simulink model "Simulation_CHB_Gridconnected"  (R2023a)
settings: Solver=ode4  StartTime=0.0  StopTime=2  FixedStep=1e-6  RelTol=1e-3
libraries: spsMosfetLib x24, spsSeriesRLCBranchLib x9, spsVoltageMeasurementLib x9, spsControlledCurrentSourceLib x6, slpidlib x5, simulink x3, eePowerMeasurement x3, spsThreePhaseVIMeasurementLib x3, spsabctodq0Lib x2, spsStairGeneratorLib x1, spsPLL3phLib x1, spsThreePhaseSeriesRLCLoadLib x1
settings Model: Creator=Vigneshwaran R  LastModifiedBy=Vigneshwaran R

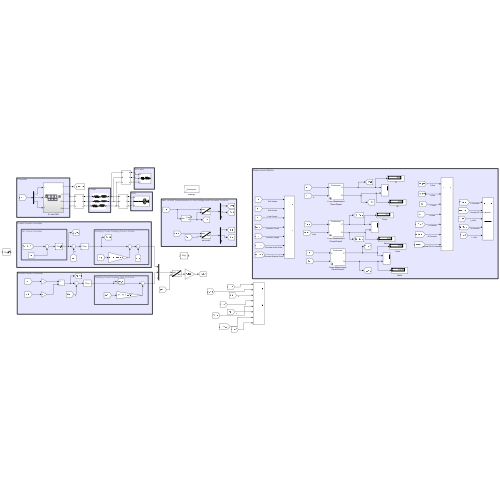
[thumbnail: Simulink's stored preview of the top-level diagram]
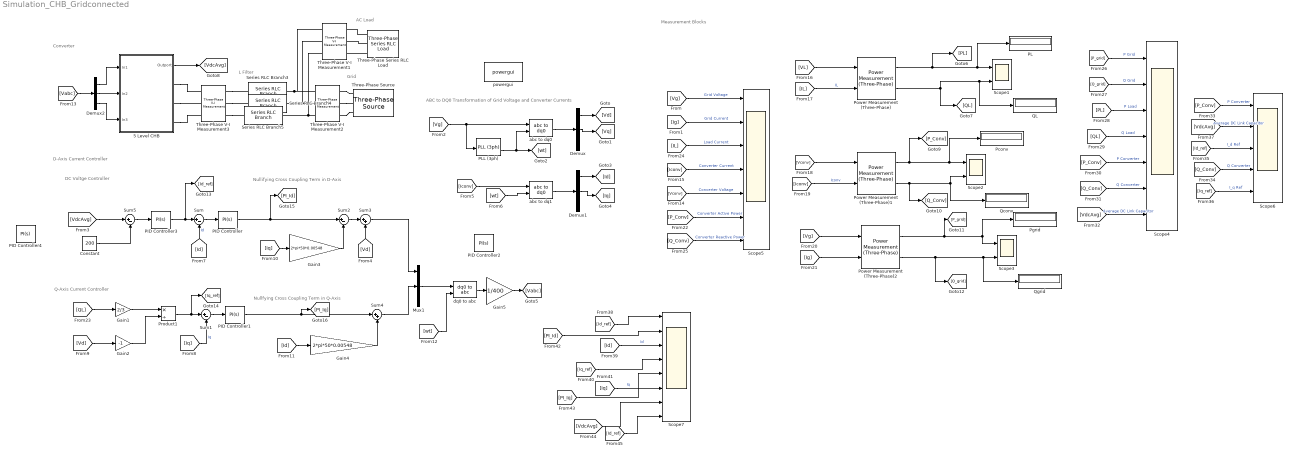
== system Simulation_CHB_Gridconnected ==
  note: Measurement Blocks
  note: L Filter
  note: D-Axis Current Controller
  note: Q-Axis Current Controller
  note: Nullfying Cross Coupling Term in Q-Axis
  note: Nullifying Cross Coupling Term in D-Axis
  note: DC Voltge Controller
  note: Grid
  note: AC Load
  note: ABC to DQ0 Transformation of Grid Voltage and Converter Currents
  note: Converter
  5 Level CHB : Subsystem
  Constant : Constant  Value=200
  Demux : Demux  Outputs=3
  Demux1 : Demux  Outputs=3
  Demux2 : Demux  Outputs=3
  Gain1 : Gain  Gain=2/3
  Gain2 : Gain  Gain=-1
  Gain3 : Gain  Gain=2*pi*50*0.00548
  Gain4 : Gain  Gain=2*pi*50*0.00548
  Gain5 : Gain  Gain=1/400
  Mux1 : Mux  Inputs=3
  PID Controller : slpidlib/PID Controller  Controller=PI  Form=Parallel  TimeDomain=Continuous-time  UseExternalTs=off  SampleTime=-1  IntegratorMethod=Forward Euler  FilterMethod=Forward Euler  ControllerParametersSource=internal  P=0.0847*400  I=1.577*400  UseKiTs=off  D=0  N=100  UseFilter=on  TunerSelectOption=Transfer Function Based (PID Tuner App)  InitialConditionSource=internal  InitialConditionForIntegrator=0  InitialConditionForFilter=0  DifferentiatorICPrevScaledInput=0  ExternalReset=none  TrackingMode=off  Kt=1  LimitOutput=off  SatLimitsSource=internal  UpperSaturationLimit=1  LowerSaturationLimit=-1  LinearizeAsGain=on  AntiWindupMode=none  Kb=1  LimitIntegrator=off  UpperIntegratorSaturationLimit=inf  LowerIntegratorSaturationLimit=-inf  POutMin=[]  POutMax=[]  IOutMin=[]  IOutMax=[]  DOutMin=[]  DOutMax=[]  NOutMin=[]  NOutMax=[]  SumOutMin=[]  SumOutMax=[]  SaturationOutMin=[]  SaturationOutMax=[]  PParamMin=[]  PParamMax=[]  IParamMin=[]  IParamMax=[]  DParamMin=[]  DParamMax=[]  NParamMin=[]  NParamMax=[]  KbParamMin=[]  KbParamMax=[]  KtParamMin=[]  KtParamMax=[]  KbOutMin=[]  KbOutMax=[]  KtOutMin=[]  KtOutMax=[]  IntegratorOutMin=[]  IntegratorOutMax=[]  FilterOutMin=[]  FilterOutMax=[]  SumI1OutMin=[]  SumI1OutMax=[]  SumI2OutMin=[]  SumI2OutMax=[]  SumI3OutMin=[]  SumI3OutMax=[]  SumI4OutMin=[]  SumI4OutMax=[]  SumDOutMin=[]  SumDOutMax=[]  DifferentiatorOutMin=[]  DifferentiatorOutMax=[]  FilterDiffOutCoefMin=[]  FilterDiffOutCoefMax=[]  ReciprocalOutMin=[]  ReciprocalOutMax=[]  SumDenOutMin=[]  SumDenOutMax=[]  SumNumOutMin=[]  SumNumOutMax=[]  DivideOutMin=[]  DivideOutMax=[]  UdiffTsProdOutMin=[]  UdiffTsProdOutMax=[]  NTsProdOutMin=[]  NTsProdOutMax=[]  UintegralTsProdOutMin=[]  UintegralTsProdOutMax=[]  UngainTsProdOutMin=[]  UngainTsProdOutMax=[]  ClampingZeroOutDataTypeStr=Inherit: Inherit via back propagation  ClampingZeroOutMin=[]  ClampingZeroOutMax=[]  FilterDenConstantOutDataTypeStr=Inherit: Inherit via back propagation  FilterDenConstantOutMin=[]  FilterDenConstantOutMax=[]  PCopyOutDataTypeStr=Inherit: Inherit via back propagation  PCopyOutMin=[]  PCopyOutMax=[]  NCopyOutDataTypeStr=Inherit: Inherit via back propagation  NCopyOutMin=[]  NCopyOutMax=[]  IntegratorContinuousStateAttributes=''  IntegratorStateMustResolveToSignalObject=off  IntegratorRTWStateStorageClass=Auto  FilterContinuousStateAttributes=''  FilterStateMustResolveToSignalObject=off  FilterRTWStateStorageClass=Auto  ParallelPVariant=InternalParameters  IdealPVariant=Disabled  IVariant=InternalParameters  DVariant=Disabled  IntegratorVariant=Continuous  SatVariant=Disabled  AWVariant=Passthrough  PCopyVariant=Disabled  TRVariant=Disabled  FdbkBlocksVariant=Forward  IdealPFdbkVariant=Disabled  SatFdbkVariant=Disabled  DerivativeFilterVariant=Disabled  NVariant=Disabled  NCopyVariant=Disabled_SignalSpec  FilterICVariant=Disabled  IntegratorICVariant=InternalICs  ExternalResetVariant=Disabled  TRSumVariant=Passthrough  SumFdbkVariant=Disabled  SumVariant=Sum_PI  TsampFilterVariant=InternalTs  TsampNgainVariant=Passthrough  TsampIntegralVariant=Disabled_SignalSpec  ExternalSaturationOutDataTypeStr=Inherit: Same as second input
  PID Controller1 : slpidlib/PID Controller  Controller=PI  Form=Parallel  TimeDomain=Continuous-time  UseExternalTs=off  SampleTime=-1  IntegratorMethod=Forward Euler  FilterMethod=Forward Euler  ControllerParametersSource=internal  P=0.0847*400  I=1.577*400  UseKiTs=off  D=0  N=100  UseFilter=on  TunerSelectOption=Transfer Function Based (PID Tuner App)  InitialConditionSource=internal  InitialConditionForIntegrator=0  InitialConditionForFilter=0  DifferentiatorICPrevScaledInput=0  ExternalReset=none  TrackingMode=off  Kt=1  LimitOutput=off  SatLimitsSource=internal  UpperSaturationLimit=1  LowerSaturationLimit=-1  LinearizeAsGain=on  AntiWindupMode=none  Kb=1  LimitIntegrator=off  UpperIntegratorSaturationLimit=inf  LowerIntegratorSaturationLimit=-inf  POutMin=[]  POutMax=[]  IOutMin=[]  IOutMax=[]  DOutMin=[]  DOutMax=[]  NOutMin=[]  NOutMax=[]  SumOutMin=[]  SumOutMax=[]  SaturationOutMin=[]  SaturationOutMax=[]  PParamMin=[]  PParamMax=[]  IParamMin=[]  IParamMax=[]  DParamMin=[]  DParamMax=[]  NParamMin=[]  NParamMax=[]  KbParamMin=[]  KbParamMax=[]  KtParamMin=[]  KtParamMax=[]  KbOutMin=[]  KbOutMax=[]  KtOutMin=[]  KtOutMax=[]  IntegratorOutMin=[]  IntegratorOutMax=[]  FilterOutMin=[]  FilterOutMax=[]  SumI1OutMin=[]  SumI1OutMax=[]  SumI2OutMin=[]  SumI2OutMax=[]  SumI3OutMin=[]  SumI3OutMax=[]  SumI4OutMin=[]  SumI4OutMax=[]  SumDOutMin=[]  SumDOutMax=[]  DifferentiatorOutMin=[]  DifferentiatorOutMax=[]  FilterDiffOutCoefMin=[]  FilterDiffOutCoefMax=[]  ReciprocalOutMin=[]  ReciprocalOutMax=[]  SumDenOutMin=[]  SumDenOutMax=[]  SumNumOutMin=[]  SumNumOutMax=[]  DivideOutMin=[]  DivideOutMax=[]  UdiffTsProdOutMin=[]  UdiffTsProdOutMax=[]  NTsProdOutMin=[]  NTsProdOutMax=[]  UintegralTsProdOutMin=[]  UintegralTsProdOutMax=[]  UngainTsProdOutMin=[]  UngainTsProdOutMax=[]  ClampingZeroOutDataTypeStr=Inherit: Inherit via back propagation  ClampingZeroOutMin=[]  ClampingZeroOutMax=[]  FilterDenConstantOutDataTypeStr=Inherit: Inherit via back propagation  FilterDenConstantOutMin=[]  FilterDenConstantOutMax=[]  PCopyOutDataTypeStr=Inherit: Inherit via back propagation  PCopyOutMin=[]  PCopyOutMax=[]  NCopyOutDataTypeStr=Inherit: Inherit via back propagation  NCopyOutMin=[]  NCopyOutMax=[]  IntegratorContinuousStateAttributes=''  IntegratorStateMustResolveToSignalObject=off  IntegratorRTWStateStorageClass=Auto  FilterContinuousStateAttributes=''  FilterStateMustResolveToSignalObject=off  FilterRTWStateStorageClass=Auto  ParallelPVariant=InternalParameters  IdealPVariant=Disabled  IVariant=InternalParameters  DVariant=Disabled  IntegratorVariant=Continuous  SatVariant=Disabled  AWVariant=Passthrough  PCopyVariant=Disabled  TRVariant=Disabled  FdbkBlocksVariant=Forward  IdealPFdbkVariant=Disabled  SatFdbkVariant=Disabled  DerivativeFilterVariant=Disabled  NVariant=Disabled  NCopyVariant=Disabled_SignalSpec  FilterICVariant=Disabled  IntegratorICVariant=InternalICs  ExternalResetVariant=Disabled  TRSumVariant=Passthrough  SumFdbkVariant=Disabled  SumVariant=Sum_PI  TsampFilterVariant=InternalTs  TsampNgainVariant=Passthrough  TsampIntegralVariant=Disabled_SignalSpec  ExternalSaturationOutDataTypeStr=Inherit: Same as second input
  PID Controller2 : slpidlib/PID Controller  Controller=PI  Form=Parallel  TimeDomain=Continuous-time  UseExternalTs=off  SampleTime=-1  IntegratorMethod=Forward Euler  FilterMethod=Forward Euler  ControllerParametersSource=internal  P=0.15  I=157.7  UseKiTs=off  D=0  N=100  UseFilter=on  TunerSelectOption=Transfer Function Based (PID Tuner App)  InitialConditionSource=internal  InitialConditionForIntegrator=0  InitialConditionForFilter=0  DifferentiatorICPrevScaledInput=0  ExternalReset=none  TrackingMode=off  Kt=1  LimitOutput=off  SatLimitsSource=internal  UpperSaturationLimit=1  LowerSaturationLimit=-1  LinearizeAsGain=on  AntiWindupMode=none  Kb=1  LimitIntegrator=off  UpperIntegratorSaturationLimit=inf  LowerIntegratorSaturationLimit=-inf  POutMin=[]  POutMax=[]  IOutMin=[]  IOutMax=[]  DOutMin=[]  DOutMax=[]  NOutMin=[]  NOutMax=[]  SumOutMin=[]  SumOutMax=[]  SaturationOutMin=[]  SaturationOutMax=[]  PParamMin=[]  PParamMax=[]  IParamMin=[]  IParamMax=[]  DParamMin=[]  DParamMax=[]  NParamMin=[]  NParamMax=[]  KbParamMin=[]  KbParamMax=[]  KtParamMin=[]  KtParamMax=[]  KbOutMin=[]  KbOutMax=[]  KtOutMin=[]  KtOutMax=[]  IntegratorOutMin=[]  IntegratorOutMax=[]  FilterOutMin=[]  FilterOutMax=[]  SumI1OutMin=[]  SumI1OutMax=[]  SumI2OutMin=[]  SumI2OutMax=[]  SumI3OutMin=[]  SumI3OutMax=[]  SumI4OutMin=[]  SumI4OutMax=[]  SumDOutMin=[]  SumDOutMax=[]  DifferentiatorOutMin=[]  DifferentiatorOutMax=[]  FilterDiffOutCoefMin=[]  FilterDiffOutCoefMax=[]  ReciprocalOutMin=[]  ReciprocalOutMax=[]  SumDenOutMin=[]  SumDenOutMax=[]  SumNumOutMin=[]  SumNumOutMax=[]  DivideOutMin=[]  DivideOutMax=[]  UdiffTsProdOutMin=[]  UdiffTsProdOutMax=[]  NTsProdOutMin=[]  NTsProdOutMax=[]  UintegralTsProdOutMin=[]  UintegralTsProdOutMax=[]  UngainTsProdOutMin=[]  UngainTsProdOutMax=[]  ClampingZeroOutDataTypeStr=Inherit: Inherit via back propagation  ClampingZeroOutMin=[]  ClampingZeroOutMax=[]  FilterDenConstantOutDataTypeStr=Inherit: Inherit via back propagation  FilterDenConstantOutMin=[]  FilterDenConstantOutMax=[]  PCopyOutDataTypeStr=Inherit: Inherit via back propagation  PCopyOutMin=[]  PCopyOutMax=[]  NCopyOutDataTypeStr=Inherit: Inherit via back propagation  NCopyOutMin=[]  NCopyOutMax=[]  IntegratorContinuousStateAttributes=''  IntegratorStateMustResolveToSignalObject=off  IntegratorRTWStateStorageClass=Auto  FilterContinuousStateAttributes=''  FilterStateMustResolveToSignalObject=off  FilterRTWStateStorageClass=Auto  ParallelPVariant=InternalParameters  IdealPVariant=Disabled  IVariant=InternalParameters  DVariant=Disabled  IntegratorVariant=Continuous  SatVariant=Disabled  AWVariant=Passthrough  PCopyVariant=Disabled  TRVariant=Disabled  FdbkBlocksVariant=Forward  IdealPFdbkVariant=Disabled  SatFdbkVariant=Disabled  DerivativeFilterVariant=Disabled  NVariant=Disabled  NCopyVariant=Disabled_SignalSpec  FilterICVariant=Disabled  IntegratorICVariant=InternalICs  ExternalResetVariant=Disabled  TRSumVariant=Passthrough  SumFdbkVariant=Disabled  SumVariant=Sum_PI  TsampFilterVariant=InternalTs  TsampNgainVariant=Passthrough  TsampIntegralVariant=Disabled_SignalSpec  ExternalSaturationOutDataTypeStr=Inherit: Same as second input
  PID Controller3 : slpidlib/PID Controller  Controller=PI  Form=Parallel  TimeDomain=Continuous-time  UseExternalTs=off  SampleTime=-1  IntegratorMethod=Forward Euler  FilterMethod=Forward Euler  ControllerParametersSource=internal  P=1*10  I=5*10  UseKiTs=off  D=0  N=100  UseFilter=on  TunerSelectOption=Transfer Function Based (PID Tuner App)  InitialConditionSource=internal  InitialConditionForIntegrator=0  InitialConditionForFilter=0  DifferentiatorICPrevScaledInput=0  ExternalReset=none  TrackingMode=off  Kt=1  LimitOutput=on  SatLimitsSource=internal  UpperSaturationLimit=200  LowerSaturationLimit=-200  LinearizeAsGain=on  AntiWindupMode=none  Kb=1  LimitIntegrator=off  UpperIntegratorSaturationLimit=inf  LowerIntegratorSaturationLimit=-inf  POutMin=[]  POutMax=[]  IOutMin=[]  IOutMax=[]  DOutMin=[]  DOutMax=[]  NOutMin=[]  NOutMax=[]  SumOutMin=[]  SumOutMax=[]  SaturationOutMin=[]  SaturationOutMax=[]  PParamMin=[]  PParamMax=[]  IParamMin=[]  IParamMax=[]  DParamMin=[]  DParamMax=[]  NParamMin=[]  NParamMax=[]  KbParamMin=[]  KbParamMax=[]  KtParamMin=[]  KtParamMax=[]  KbOutMin=[]  KbOutMax=[]  KtOutMin=[]  KtOutMax=[]  IntegratorOutMin=[]  IntegratorOutMax=[]  FilterOutMin=[]  FilterOutMax=[]  SumI1OutMin=[]  SumI1OutMax=[]  SumI2OutMin=[]  SumI2OutMax=[]  SumI3OutMin=[]  SumI3OutMax=[]  SumI4OutMin=[]  SumI4OutMax=[]  SumDOutMin=[]  SumDOutMax=[]  DifferentiatorOutMin=[]  DifferentiatorOutMax=[]  FilterDiffOutCoefMin=[]  FilterDiffOutCoefMax=[]  ReciprocalOutMin=[]  ReciprocalOutMax=[]  SumDenOutMin=[]  SumDenOutMax=[]  SumNumOutMin=[]  SumNumOutMax=[]  DivideOutMin=[]  DivideOutMax=[]  UdiffTsProdOutMin=[]  UdiffTsProdOutMax=[]  NTsProdOutMin=[]  NTsProdOutMax=[]  UintegralTsProdOutMin=[]  UintegralTsProdOutMax=[]  UngainTsProdOutMin=[]  UngainTsProdOutMax=[]  ClampingZeroOutDataTypeStr=Inherit: Inherit via back propagation  ClampingZeroOutMin=[]  ClampingZeroOutMax=[]  FilterDenConstantOutDataTypeStr=Inherit: Inherit via back propagation  FilterDenConstantOutMin=[]  FilterDenConstantOutMax=[]  PCopyOutDataTypeStr=Inherit: Inherit via back propagation  PCopyOutMin=[]  PCopyOutMax=[]  NCopyOutDataTypeStr=Inherit: Inherit via back propagation  NCopyOutMin=[]  NCopyOutMax=[]  IntegratorContinuousStateAttributes=''  IntegratorStateMustResolveToSignalObject=off  IntegratorRTWStateStorageClass=Auto  FilterContinuousStateAttributes=''  FilterStateMustResolveToSignalObject=off  FilterRTWStateStorageClass=Auto  ParallelPVariant=InternalParameters  IdealPVariant=Disabled  IVariant=InternalParameters  DVariant=Disabled  IntegratorVariant=Continuous  SatVariant=Enabled  AWVariant=Passthrough  PCopyVariant=Disabled  TRVariant=Disabled  FdbkBlocksVariant=Forward  IdealPFdbkVariant=Disabled  SatFdbkVariant=Disabled  DerivativeFilterVariant=Disabled  NVariant=Disabled  NCopyVariant=Disabled_SignalSpec  FilterICVariant=Disabled  IntegratorICVariant=InternalICs  ExternalResetVariant=Disabled  TRSumVariant=Passthrough  SumFdbkVariant=Disabled  SumVariant=Sum_PI  TsampFilterVariant=InternalTs  TsampNgainVariant=Passthrough  TsampIntegralVariant=Disabled_SignalSpec  ExternalSaturationOutDataTypeStr=Inherit: Same as second input
  PID Controller4 : slpidlib/PID Controller  Controller=PI  Form=Parallel  TimeDomain=Continuous-time  UseExternalTs=off  SampleTime=-1  IntegratorMethod=Forward Euler  FilterMethod=Forward Euler  ControllerParametersSource=internal  P=1  I=5  UseKiTs=off  D=0  N=100  UseFilter=on  TunerSelectOption=Transfer Function Based (PID Tuner App)  InitialConditionSource=internal  InitialConditionForIntegrator=0  InitialConditionForFilter=0  DifferentiatorICPrevScaledInput=0  ExternalReset=none  TrackingMode=off  Kt=1  LimitOutput=on  SatLimitsSource=internal  UpperSaturationLimit=200  LowerSaturationLimit=-200  LinearizeAsGain=on  AntiWindupMode=none  Kb=1  LimitIntegrator=off  UpperIntegratorSaturationLimit=inf  LowerIntegratorSaturationLimit=-inf  POutMin=[]  POutMax=[]  IOutMin=[]  IOutMax=[]  DOutMin=[]  DOutMax=[]  NOutMin=[]  NOutMax=[]  SumOutMin=[]  SumOutMax=[]  SaturationOutMin=[]  SaturationOutMax=[]  PParamMin=[]  PParamMax=[]  IParamMin=[]  IParamMax=[]  DParamMin=[]  DParamMax=[]  NParamMin=[]  NParamMax=[]  KbParamMin=[]  KbParamMax=[]  KtParamMin=[]  KtParamMax=[]  KbOutMin=[]  KbOutMax=[]  KtOutMin=[]  KtOutMax=[]  IntegratorOutMin=[]  IntegratorOutMax=[]  FilterOutMin=[]  FilterOutMax=[]  SumI1OutMin=[]  SumI1OutMax=[]  SumI2OutMin=[]  SumI2OutMax=[]  SumI3OutMin=[]  SumI3OutMax=[]  SumI4OutMin=[]  SumI4OutMax=[]  SumDOutMin=[]  SumDOutMax=[]  DifferentiatorOutMin=[]  DifferentiatorOutMax=[]  FilterDiffOutCoefMin=[]  FilterDiffOutCoefMax=[]  ReciprocalOutMin=[]  ReciprocalOutMax=[]  SumDenOutMin=[]  SumDenOutMax=[]  SumNumOutMin=[]  SumNumOutMax=[]  DivideOutMin=[]  DivideOutMax=[]  UdiffTsProdOutMin=[]  UdiffTsProdOutMax=[]  NTsProdOutMin=[]  NTsProdOutMax=[]  UintegralTsProdOutMin=[]  UintegralTsProdOutMax=[]  UngainTsProdOutMin=[]  UngainTsProdOutMax=[]  ClampingZeroOutDataTypeStr=Inherit: Inherit via back propagation  ClampingZeroOutMin=[]  ClampingZeroOutMax=[]  FilterDenConstantOutDataTypeStr=Inherit: Inherit via back propagation  FilterDenConstantOutMin=[]  FilterDenConstantOutMax=[]  PCopyOutDataTypeStr=Inherit: Inherit via back propagation  PCopyOutMin=[]  PCopyOutMax=[]  NCopyOutDataTypeStr=Inherit: Inherit via back propagation  NCopyOutMin=[]  NCopyOutMax=[]  IntegratorContinuousStateAttributes=''  IntegratorStateMustResolveToSignalObject=off  IntegratorRTWStateStorageClass=Auto  FilterContinuousStateAttributes=''  FilterStateMustResolveToSignalObject=off  FilterRTWStateStorageClass=Auto  ParallelPVariant=InternalParameters  IdealPVariant=Disabled  IVariant=InternalParameters  DVariant=Disabled  IntegratorVariant=Continuous  SatVariant=Enabled  AWVariant=Passthrough  PCopyVariant=Disabled  TRVariant=Disabled  FdbkBlocksVariant=Forward  IdealPFdbkVariant=Disabled  SatFdbkVariant=Disabled  DerivativeFilterVariant=Disabled  NVariant=Disabled  NCopyVariant=Disabled_SignalSpec  FilterICVariant=Disabled  IntegratorICVariant=InternalICs  ExternalResetVariant=Disabled  TRSumVariant=Passthrough  SumFdbkVariant=Disabled  SumVariant=Sum_PI  TsampFilterVariant=InternalTs  TsampNgainVariant=Passthrough  TsampIntegralVariant=Disabled_SignalSpec  ExternalSaturationOutDataTypeStr=Inherit: Same as second input
  PL : Display
  PLL (3ph) : spsPLL3phLib/PLL (3ph)  Fmin=45  Par_Init=[0, 50]  ParK=[180, 3200, 1]  TcD=1e-4  MaxRateChangeFreq=12  FilterCutOffFreq=25  Ts=0  AGC=on
  Pconv : Display
  Pgrid : Display
  Power Measurement (Three-Phase) : eePowerMeasurement/Power Measurement (Three-Phase)  LabelModeActiveChoice=Continuous  F=50  K=[1]  Seq=Positive  Ts=0
  Power Measurement (Three-Phase)1 : eePowerMeasurement/Power Measurement (Three-Phase)  LabelModeActiveChoice=Continuous  F=50  K=[1]  Seq=Positive  Ts=0
  Power Measurement (Three-Phase)2 : eePowerMeasurement/Power Measurement (Three-Phase)  LabelModeActiveChoice=Continuous  F=50  K=[1]  Seq=Positive  Ts=0
  Product1 : Product  Inputs=*/
  QL : Display
  Qconv : Display
  Qgrid : Display
  Scope1 : Scope  NumInputPorts=2
  Scope2 : Scope  NumInputPorts=2
  Scope3 : Scope  NumInputPorts=2
  Scope4 : Scope  NumInputPorts=7
  Scope5 : Scope  NumInputPorts=7
  Scope6 : Scope  NumInputPorts=5
  Scope7 : Scope  NumInputPorts=8
  Series RLC Branch3 : spsSeriesRLCBranchLib/Series RLC Branch  LConnTagsString=__new0  RConnTagsString=__new0  BranchType=RL  Resistance=0.1  Inductance=5.48e-3  SetiL0=off  InitialCurrent=0  Capacitance=1e-6  Setx0=off  InitialVoltage=0  Measurements=None
  Series RLC Branch4 : spsSeriesRLCBranchLib/Series RLC Branch  LConnTagsString=__new0  RConnTagsString=__new0  BranchType=RL  Resistance=0.1  Inductance=5.48e-3  SetiL0=off  InitialCurrent=0  Capacitance=1e-6  Setx0=off  InitialVoltage=0  Measurements=None
  Series RLC Branch5 : spsSeriesRLCBranchLib/Series RLC Branch  LConnTagsString=__new0  RConnTagsString=__new0  BranchType=RL  Resistance=0.1  Inductance=5.48e-3  SetiL0=off  InitialCurrent=0  Capacitance=1e-6  Setx0=off  InitialVoltage=0  Measurements=None
  Sum{,1..2,5} (4 alike) : Sum  Inputs=|+-
  Sum3 : Sum  Inputs=|++
  Sum4 : Sum  Inputs=|++
  Three-Phase Series RLC Load : spsThreePhaseSeriesRLCLoadLib/Three-Phase Series RLC Load  LConnTagsString=A|B|C  Configuration=Y (grounded)  NominalVoltage=415  Vabc=[1e3 1e3 1e3]  Vabcp=[1e3 1e3 1e3]  NominalFrequency=50  UnbalancedPower=off  ActivePower=4e3  InductivePower=4e3  CapacitivePower=0  Pabc=[10e3 9e3 11e3]  QLabc=[100 90 110]  QCabc=[100 90 110]  Pabcp=[10e3 9e3 11e3]  QLabcp=[100 90 110]  QCabcp=[100 90 110]  Measurements=None  LoadType=constant Z
  Three-Phase V-I Measurement1 : spsThreePhaseVIMeasurementLib/Three-Phase V-I Measurement  VoltageMeasurement=phase-to-ground  SetLabelV=on  LabelV=VL  Vpu=off  VpuLL=off  CurrentMeasurement=yes  SetLabelI=on  LabelI=IL  Ipu=off  Pbase=100e6  Vbase=500e3  OutputType=Complex  PhasorSimulation=off  PSBequivalent=0
  Three-Phase V-I Measurement2 : spsThreePhaseVIMeasurementLib/Three-Phase V-I Measurement  VoltageMeasurement=phase-to-ground  SetLabelV=on  LabelV=Vg  Vpu=off  VpuLL=off  CurrentMeasurement=yes  SetLabelI=on  LabelI=Ig  Ipu=off  Pbase=100e6  Vbase=500e3  OutputType=Complex  PhasorSimulation=off  PSBequivalent=0
  Three-Phase V-I Measurement3 : spsThreePhaseVIMeasurementLib/Three-Phase V-I Measurement  VoltageMeasurement=phase-to-ground  SetLabelV=on  LabelV=Vconv  Vpu=off  VpuLL=off  CurrentMeasurement=yes  SetLabelI=on  LabelI=Iconv  Ipu=off  Pbase=100e6  Vbase=500e3  OutputType=Complex  PhasorSimulation=off  PSBequivalent=0
  Three-Phase Source : spsThreePhaseSourceLib/Three-Phase Source  InternalConnection=Yg  VoltagePhases=off  Voltage=415  PhaseAngle=0  Voltage_phases=[25e3 25e3 25e3]/sqrt(3)  PhaseAngles_phases=[0 -120 +120]  Frequency=50  NonIdealSource=off  SpecifyImpedance=off  Resistance=0  Inductance=0  ShortCircuitLevel=100e6  BaseVoltage=25e3  XRratio=7  BusType=swing  Pref=10e3  Qref=0  Prefabc=[10e3, 10e3, 10e3]  Qrefabc=[0, 0, 0]  Qmin=-inf  Qmax=inf
  abc to dq0 : spsabctodq0Lib/abc to dq0  Alignment=90 degrees behind phase A axis
  abc to dq1 : spsabctodq0Lib/abc to dq0  Alignment=90 degrees behind phase A axis
  dq0 to abc : spsdq0toabcLib/dq0 to abc  Alignment=90 degrees behind phase A axis
  powergui : sps_lib/powergui  Priority=1  SimulationMode=Continuous  SampleTime=50e-6  frequency=60  Iterations=50  frequencyindice=0  Pbase=100e6  ErrMax=1e-4  UnitsV=kV  UnitsW=MW  buscounter=0  FunctionMessages=off  echomessages=off  EnableUseOfTLC=off  CurrentSourceSwitches=off  DisableSnubberDevices=off  DisableRonSwitches=off  DisableVfSwitches=off  DisplayEquations=off  AutomaticDiscreteSolvers=off  SolverType=Tustin/Backward Euler (TBE)  Interpol=off  ExternalGateDelay=off  methode=off  Ts=100  x0status=blocks  SPID=on  SwTol=0  HookPort=off  NonlinearTolerance=1e-4  nMaxIteration=100  ContinueOnMaxIteration=off  RestoreLinks=warning  ResistiveCurrentMeasurement=off  Frange=[0:2:500]  Ylog=off  Xlog=on  ShowGrid=off  save=off  variable=ZData  structure=0  ZoomFFT=off  StartTime=0.0  cycles=1  DisplayStyle=1  fundamental=60  FreqAxis=off  MaxFrequency=1000  frequencyindicesteady=1  RmsSteady=1  display=off
  wires:
  [Vg] -> PLL (3ph)/1, abc to dq0/1
  PLL (3ph)/2 -> abc to dq0/2, [wt]
  abc to dq0/1 -> Demux/1
  Demux/1 -> [Vd]
  Demux/2 -> [Vq]
  Demux1/2 -> [Iq]
  Demux1/1 -> [Id]
  abc to dq1/1 -> Demux1/1
  [Iconv] -> abc to dq1/1
  [wt] -> abc to dq1/2
  [Vd] -> Gain2/1
  Gain1/1 -> Product1/1
  PID Controller3/1 -> [Id_ref], Sum/1
  Product1/1 -> [Iq_ref], Sum1/1
  [Id] -> Sum/2  "Id"
  [Iq] -> Sum1/2  "Iq"
  Gain2/1 -> Product1/2
  Sum/1 -> PID Controller/1
  Sum1/1 -> PID Controller1/1
  PID Controller/1 -> [PI_Id], Sum2/1
  [Iq] -> Gain3/1
  Gain3/1 -> Sum2/2
  Sum2/1 -> Sum3/1
  [Vd] -> Sum3/2
  PID Controller1/1 -> [PI_Iq], Sum4/1
  Gain4/1 -> Sum4/2
  [Id] -> Gain4/1
  Sum3/1 -> Mux1/1
  Mux1/1 -> dq0 to abc/1
  [wt] -> dq0 to abc/2
  dq0 to abc/1 -> Gain5/1
  [Vabc] -> Demux2/1
  Demux2/1 -> 5 Level CHB/1(In1)
  Demux2/2 -> 5 Level CHB/2(In2)
  Demux2/3 -> 5 Level CHB/3(In3)
  Sum4/1 -> Mux1/2
  Gain5/1 -> [Vabc]
  Power Measurement (Three-Phase)/1 -> [PL], PL/1, Scope1/1
  Power Measurement (Three-Phase)/2 -> [QL], QL/1, Scope1/2
  [VL] -> Power Measurement (Three-Phase)/1
  [IL] -> Power Measurement (Three-Phase)/2  "IL"
  Power Measurement (Three-Phase)1/2 -> Scope2/2, Qconv/1, [Q_Conv]
  Power Measurement (Three-Phase)1/1 -> Scope2/1, Pconv/1, [P_Conv]
  [Vconv] -> Power Measurement (Three-Phase)1/1
  [Iconv] -> Power Measurement (Three-Phase)1/2  "Iconv"
  [Ig] -> Power Measurement (Three-Phase)2/2
  Power Measurement (Three-Phase)2/1 -> [P_grid], Scope3/1, Pgrid/1
  Power Measurement (Three-Phase)2/2 -> Qgrid/1, Scope3/2, [Q_grid]
  [QL] -> Gain1/1
  [Vg] -> Power Measurement (Three-Phase)2/1
  5 Level CHB/1(Outport) -> [VdcAvg]
  [VdcAvg] -> Sum5/1
  Constant/1 -> Sum5/2
  Sum5/1 -> PID Controller3/1
  [Vg] -> Scope5/1  "Grid Voltage"
  [Vconv] -> Scope5/5  "Converter Voltage"
  [Ig] -> Scope5/2  "Grid Current"
  [IL] -> Scope5/3  "Load Current"
  [Iconv] -> Scope5/4  "Converter Current"
  [P_Conv] -> Scope5/6  "Converter Active Power"
  [Q_Conv] -> Scope5/7  "Converter Reactive Power"
  [P_grid] -> Scope4/1  "P Grid"
  [Q_grid] -> Scope4/2  "Q Grid"
  [PL] -> Scope4/3  "P Load"
  [QL] -> Scope4/4  "Q Load"
  [P_Conv] -> Scope4/5  "P Converter"
  [Q_Conv] -> Scope4/6  "Q Converter"
  [VdcAvg] -> Scope4/7  "Average DC Link Capacitor"
  [P_Conv] -> Scope6/1  "P Converter"
  [Q_Conv] -> Scope6/4  "Q Converter"
  [Id_ref] -> Scope6/3  "I_d Ref"
  [Iq_ref] -> Scope6/5  "I_q Ref"
  [VdcAvg] -> Scope6/2  "Average DC Link Capacitor"
  [Id_ref] -> Scope7/1
  [Id] -> Scope7/3  "Id"
  [Iq_ref] -> Scope7/4
  [Iq] -> Scope7/6  "Iq"
  [PI_Id] -> Scope7/2
  [PI_Iq] -> Scope7/5
  [VdcAvg] -> Scope7/7
  [Id_ref] -> Scope7/8
  connections:
  Three-Phase Series RLC Load/LConn1 -- Three-Phase V-I Measurement1/RConn1
  Three-Phase Series RLC Load/LConn2 -- Three-Phase V-I Measurement1/RConn2
  Three-Phase Series RLC Load/LConn3 -- Three-Phase V-I Measurement1/RConn3
  Three-Phase V-I Measurement1/LConn3 -- Three-Phase V-I Measurement2/RConn3 -- Series RLC Branch5/RConn1
  5 Level CHB/RConn1 -- Three-Phase V-I Measurement3/LConn1
  Three-Phase V-I Measurement3/RConn1 -- Series RLC Branch3/LConn1
  5 Level CHB/RConn2 -- Three-Phase V-I Measurement3/LConn2
  Three-Phase V-I Measurement3/RConn2 -- Series RLC Branch4/LConn1
  5 Level CHB/RConn3 -- Three-Phase V-I Measurement3/LConn3
  Three-Phase V-I Measurement3/RConn3 -- Series RLC Branch5/LConn1
  Three-Phase V-I Measurement2/LConn1 -- Three-Phase Source/RConn1
  Three-Phase V-I Measurement2/LConn2 -- Three-Phase Source/RConn2
  Three-Phase V-I Measurement2/LConn3 -- Three-Phase Source/RConn3
  Series RLC Branch3/RConn1 -- Three-Phase V-I Measurement2/RConn1 -- Three-Phase V-I Measurement1/LConn1
  Series RLC Branch4/RConn1 -- Three-Phase V-I Measurement2/RConn2 -- Three-Phase V-I Measurement1/LConn2

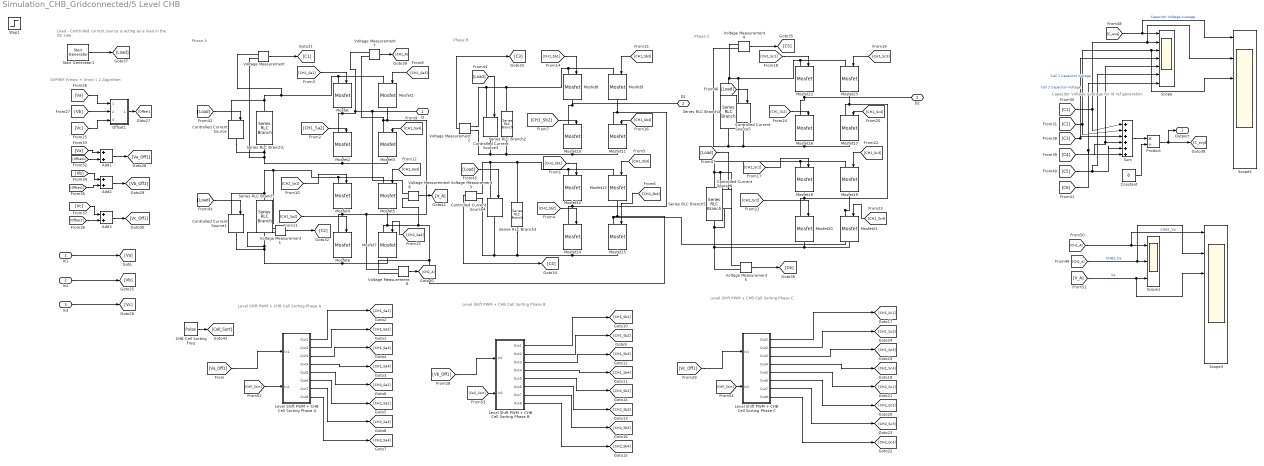
== system Simulation_CHB_Gridconnected/5 Level CHB ==
  note: Level Shift PWM + CHB Cell Sorting Phase C
  note: Level Shift PWM + CHB Cell Sorting Phase B
  note: Capacitor Voltage Average for Id ref generation
  note: Load - Controlled current source is acting
      | as a load in the DC side.
  note: SVPWM (Vmax + Vmin) / 2 Algorithm
  note: Phase C
  note: Phase B
  note: Phase A
  note: Level Shift PWM + CHB Cell Sorting Phase A
  In1 : Inport
  In2 : Inport  Port=2
  In3 : Inport  Port=3
  Add1 : Sum
  Add2 : Sum
  Add3 : Sum
  CHB Cell Sorting Freq : DiscretePulseGenerator  PulseType=Time based  Period=1/4000  PulseWidth=50
  Constant : Constant  Value=6
  Controlled Current Source{,1,3..6} (6 alike) : spsControlledCurrentSourceLib/Controlled Current Source  Initialize=on  Source_Type=DC  Amplitude=0  Phase=0  Frequency=0  Measurements=None
  Level Shift PWM + CHB Cell Sorting Phase A : Subsystem
  Level Shift PWM + CHB Cell Sorting Phase B : Subsystem
  Level Shift PWM + CHB Cell Sorting Phase C : Subsystem
  Mosfet{,1..23} (24 alike) : spsMosfetLib/Mosfet  Ron=0.1  Lon=0  Rd=0.01  Vfd=0  IC=0  Rs=1e5  Cs=inf  Measurements=off
  Offset1 : Subsystem
  Product : Product  Inputs=*/
  Scope : Scope  NumInputPorts=7
  Scope1 : Scope  NumInputPorts=3
  Scope3 : Scope  NumInputPorts=7
  Scope5 : Scope  NumInputPorts=7
  Series RLC Branch{,1..5} (6 alike) : spsSeriesRLCBranchLib/Series RLC Branch  LConnTagsString=__new0  RConnTagsString=__new0  BranchType=C  Resistance=1  Inductance=1e-3  SetiL0=off  InitialCurrent=0  Capacitance=5600e-6  Setx0=on  InitialVoltage=200  Measurements=None
  Stair Generator1 : spsStairGeneratorLib/Stair Generator  t=[0, 0.7, 1.5]  e=[0, 5, 0]  Ts=0
  Step1 : Step  Time=0.7  After=5  SampleTime=0
  Sum : Sum  Inputs=|++++++
  Voltage Measurement{,1..8} (9 alike) : spsVoltageMeasurementLib/Voltage Measurement  PhasorSimulation=off  OutputType=Complex  PSBequivalent=0
  D : PMIOPort  Side=Right
  D1 : PMIOPort  Port=2  Side=Right
  D2 : PMIOPort  Port=3  Side=Right
  Outport : Outport
  wires:
  Level Shift PWM + CHB Cell Sorting Phase A/5(Out5) -> [CH2_Sa1]
  Level Shift PWM + CHB Cell Sorting Phase B/2(Out2) -> [CH1_Sb2]
  [CH2_Sb1] -> Mosfet12/1
  Level Shift PWM + CHB Cell Sorting Phase A/6(Out6) -> [CH2_Sa2]
  [CH1_Sb3] -> Mosfet9/1
  [CH1_Sb2] -> Mosfet10/1
  Level Shift PWM + CHB Cell Sorting Phase A/4(Out4) -> [CH1_Sa4]
  [CH1_Sa1] -> Mosfet/1
  [CH1_Sb1] -> Mosfet8/1
  Level Shift PWM + CHB Cell Sorting Phase A/7(Out7) -> [CH2_Sa3]
  Level Shift PWM + CHB Cell Sorting Phase B/3(Out3) -> [CH1_Sb3]
  Level Shift PWM + CHB Cell Sorting Phase C/3(Out3) -> [CH1_Sc3]
  [Vc_Off1] -> Level Shift PWM + CHB Cell Sorting Phase C/1(In1)
  [CH2_Sc4] -> Mosfet21/1
  Level Shift PWM + CHB Cell Sorting Phase B/5(Out5) -> [CH2_Sb1]
  [CH2_Sa1] -> Mosfet4/1
  [CH1_Sa3] -> Mosfet1/1
  Level Shift PWM + CHB Cell Sorting Phase C/5(Out5) -> [CH2_Sc1]
  [CH1_Sc4] -> Mosfet17/1
  [CH1_Sa2] -> Mosfet2/1
  [CH1_Sa4] -> Mosfet3/1
  [CH2_Sa3] -> Mosfet5/1
  Level Shift PWM + CHB Cell Sorting Phase A/8(Out8) -> [CH2_Sa4]
  [CH2_Sa4] -> Mosfet7/1
  Level Shift PWM + CHB Cell Sorting Phase B/6(Out6) -> [CH2_Sb2]
  Level Shift PWM + CHB Cell Sorting Phase A/3(Out3) -> [CH1_Sa3]
  Level Shift PWM + CHB Cell Sorting Phase A/2(Out2) -> [CH1_Sa2]
  Level Shift PWM + CHB Cell Sorting Phase B/7(Out7) -> [CH2_Sb3]
  Level Shift PWM + CHB Cell Sorting Phase B/1(Out1) -> [CH1_Sb1]
  [CH1_Sc3] -> Mosfet23/1
  Level Shift PWM + CHB Cell Sorting Phase C/7(Out7) -> [CH2_Sc3]
  Level Shift PWM + CHB Cell Sorting Phase C/8(Out8) -> [CH2_Sc4]
  [CH2_Sc2] -> Mosfet20/1
  Level Shift PWM + CHB Cell Sorting Phase A/1(Out1) -> [CH1_Sa1]
  [CH2_Sb2] -> Mosfet14/1
  Level Shift PWM + CHB Cell Sorting Phase B/4(Out4) -> [CH1_Sb4]
  Level Shift PWM + CHB Cell Sorting Phase C/2(Out2) -> [CH1_Sc2]
  [CH2_Sa2] -> Mosfet6/1
  [CH1_Sc1] -> Mosfet22/1
  Level Shift PWM + CHB Cell Sorting Phase C/1(Out1) -> [CH1_Sc1]
  Level Shift PWM + CHB Cell Sorting Phase C/4(Out4) -> [CH1_Sc4]
  [CH2_Sb3] -> Mosfet13/1
  Level Shift PWM + CHB Cell Sorting Phase C/6(Out6) -> [CH2_Sc2]
  Level Shift PWM + CHB Cell Sorting Phase B/8(Out8) -> [CH2_Sb4]
  [CH2_Sc1] -> Mosfet18/1
  [CH1_Sb4] -> Mosfet11/1
  [CH1_Sc2] -> Mosfet16/1
  [CH2_Sc3] -> Mosfet19/1
  [CH2_Sb4] -> Mosfet15/1
  Add2/1 -> [Vb_Off1]
  [Vb] -> Add2/1
  [Offset1] -> Add2/2
  [Offset1] -> Add1/2
  [Vc] -> Add3/1
  Add3/1 -> [Vc_Off1]
  Offset1/1(Out1) -> [Offset1]
  [Offset1] -> Add3/2
  [Vb] -> Offset1/2(In2)
  [Va] -> Offset1/1(In1)
  [Va] -> Add1/1
  Add1/1 -> [Va_Off1]
  [Vc] -> Offset1/3(In3)
  [Vb_Off1] -> Level Shift PWM + CHB Cell Sorting Phase B/1(In1)
  [Va_Off1] -> Level Shift PWM + CHB Cell Sorting Phase A/1(In1)
  In2/1 -> [Vb]
  In1/1 -> [Va]
  In3/1 -> [Vc]
  Voltage Measurement/1 -> [C1]
  Voltage Measurement1/1 -> [C2]
  Voltage Measurement2/1 -> [C3]
  Voltage Measurement3/1 -> [C4]
  Voltage Measurement4/1 -> [C5]
  Voltage Measurement5/1 -> [C6]
  [C2] -> Scope5/3, Scope/3, Sum/2  "Cell 2 Capacitor Voltage"
  [C3] -> Scope/4, Sum/3
  [C4] -> Scope/5, Sum/4
  [C5] -> Scope/6, Sum/5
  [C6] -> Scope/7, Sum/6
  Sum/1 -> Product/1
  Constant/1 -> Product/2
  Product/1 -> [C_avg], Outport/1
  [C1] -> Scope5/2, Scope/2, Sum/1  "Cell 1 Capacitor Voltage"
  Stair Generator1/1 -> [Load]
  [Load] -> Controlled Current Source/1
  [Load] -> Controlled Current Source1/1
  [Load] -> Controlled Current Source3/1
  [Load] -> Controlled Current Source4/1
  [Load] -> Controlled Current Source5/1
  [Load] -> Controlled Current Source6/1
  [C_avg] -> Scope5/1, Scope/1  "Capacitor Voltage Average"
  Voltage Measurement7/1 -> [CH1_A]
  Voltage Measurement6/1 -> [CH2_A]
  [CH1_A] -> Scope3/1, Scope1/1  "CHB1_Va"
  [CH2_A] -> Scope3/2, Scope1/2  "CHB2_Va"
  Voltage Measurement8/1 -> [V_A]
  [V_A] -> Scope3/3, Scope1/3  "Va"
  CHB Cell Sorting Freq/1 -> [Cell_Sort]
  [Cell_Sort] -> Level Shift PWM + CHB Cell Sorting Phase A/2(In2)
  [Cell_Sort] -> Level Shift PWM + CHB Cell Sorting Phase B/2(In2)
  [Cell_Sort] -> Level Shift PWM + CHB Cell Sorting Phase C/2(In2)
  connections:
  Mosfet4/LConn1 -- Voltage Measurement1/LConn1 -- Controlled Current Source1/LConn1 -- Series RLC Branch/LConn1 -- Mosfet5/LConn1
  Mosfet/RConn1 -- Mosfet2/LConn1 -- Voltage Measurement7/LConn1 -- D/RConn1 -- Voltage Measurement8/LConn1
  Mosfet22/RConn1 -- Mosfet16/LConn1 -- D2/RConn1
  Mosfet9/RConn1 -- Mosfet11/LConn1 -- Mosfet14/LConn1 -- Mosfet12/RConn1
  Mosfet11/RConn1 -- Voltage Measurement2/LConn2 -- Controlled Current Source3/RConn1 -- Series RLC Branch2/RConn1 -- Mosfet10/RConn1
  Mosfet16/RConn1 -- Controlled Current Source5/RConn1 -- Voltage Measurement4/LConn2 -- Series RLC Branch4/RConn1 -- Mosfet17/RConn1
  Mosfet19/RConn1 -- Mosfet13/RConn1 -- Voltage Measurement8/LConn2 -- Mosfet5/RConn1 -- Mosfet7/LConn1 -- Voltage Measurement6/LConn2 -- Mosfet15/LConn1 -- Mosfet21/LConn1
  Mosfet15/RConn1 -- Controlled Current Source4/RConn1 -- Voltage Measurement3/LConn2 -- Series RLC Branch3/RConn1 -- Mosfet14/RConn1
  Mosfet9/LConn1 -- Voltage Measurement2/LConn1 -- Controlled Current Source3/LConn1 -- Series RLC Branch2/LConn1 -- Mosfet8/LConn1
  Mosfet1/RConn1 -- Mosfet3/LConn1 -- Voltage Measurement7/LConn2 -- Voltage Measurement6/LConn1 -- Mosfet6/LConn1 -- Mosfet4/RConn1
  Mosfet/LConn1 -- Controlled Current Source/LConn1 -- Series RLC Branch1/LConn1 -- Voltage Measurement/LConn1 -- Mosfet1/LConn1
  Mosfet22/LConn1 -- Controlled Current Source5/LConn1 -- Voltage Measurement4/LConn1 -- Series RLC Branch4/LConn1 -- Mosfet23/LConn1
  Mosfet17/LConn1 -- Mosfet23/RConn1 -- Mosfet20/LConn1 -- Mosfet18/RConn1
  Mosfet8/RConn1 -- Mosfet10/LConn1 -- D1/RConn1
  Mosfet6/RConn1 -- Controlled Current Source1/RConn1 -- Voltage Measurement1/LConn2 -- Series RLC Branch/RConn1 -- Mosfet7/RConn1
  Mosfet20/RConn1 -- Controlled Current Source6/RConn1 -- Series RLC Branch5/RConn1 -- Voltage Measurement5/LConn2 -- Mosfet21/RConn1
  Voltage Measurement/LConn2 -- Controlled Current Source/RConn1 -- Series RLC Branch1/RConn1 -- Mosfet2/RConn1 -- Mosfet3/RConn1
  Mosfet12/LConn1 -- Controlled Current Source4/LConn1 -- Voltage Measurement3/LConn1 -- Series RLC Branch3/LConn1 -- Mosfet13/LConn1
  Voltage Measurement5/LConn1 -- Mosfet18/LConn1 -- Mosfet19/LConn1 -- Series RLC Branch5/LConn1 -- Controlled Current Source6/LConn1

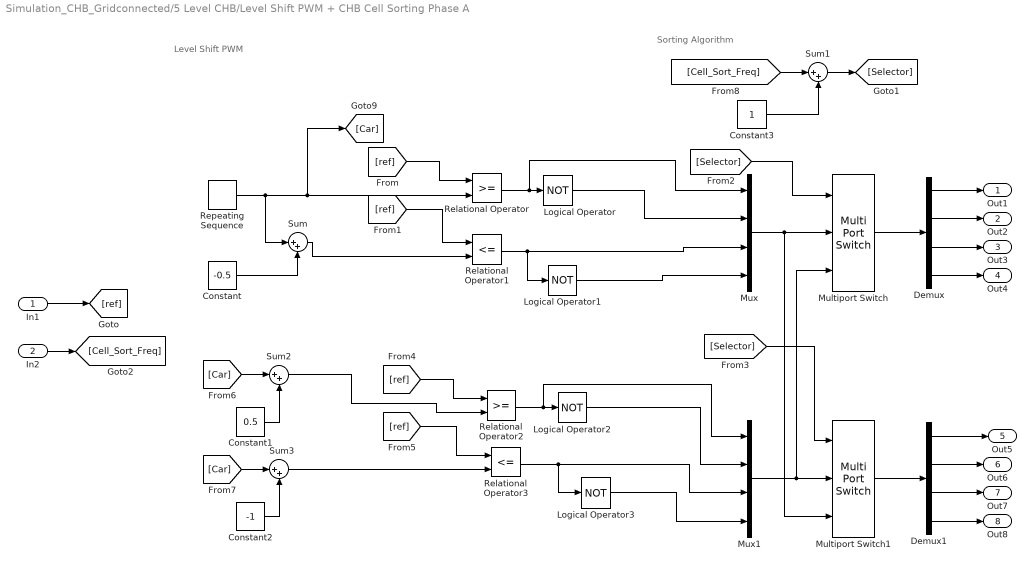
== system Simulation_CHB_Gridconnected/5 Level CHB/Level Shift PWM + CHB Cell Sorting Phase A ==
  note: Level Shift PWM
  note: Sorting Algorithm
  In1 : Inport
  In2 : Inport  Port=2
  Constant : Constant  Value=-0.5
  Constant1 : Constant  Value=0.5
  Constant2 : Constant  Value=-1
  Constant3 : Constant
  Demux : Demux
  Demux1 : Demux
  Logical Operator{,1..3} (4 alike) : Logic  Operator=NOT  AllPortsSameDT=off  OutDataTypeStr=boolean
  Multiport Switch : MultiPortSwitch  Inputs=2  SaturateOnIntegerOverflow=off  InputSameDT=off
  Multiport Switch1 : MultiPortSwitch  Inputs=2  SaturateOnIntegerOverflow=off  InputSameDT=off
  Mux : Mux
  Mux1 : Mux
  Relational Operator : RelationalOperator  OutDataTypeStr=boolean  RndMeth=Simplest  InputSameDT=off
  Relational Operator1 : RelationalOperator  Operator=<=  OutDataTypeStr=boolean  RndMeth=Simplest  InputSameDT=off
  Relational Operator2 : RelationalOperator  OutDataTypeStr=boolean  RndMeth=Simplest  InputSameDT=off
  Relational Operator3 : RelationalOperator  Operator=<=  OutDataTypeStr=boolean  RndMeth=Simplest  InputSameDT=off
  Repeating Sequence : simulink/Sources/Repeating Sequence  rep_seq_t=[0 0.5 1]/10000  rep_seq_y=[0 0.5 0]
  Sum{,1..3} (4 alike) : Sum  Inputs=|++
  Out1 : Outport
  Out2 : Outport  Port=2
  Out3 : Outport  Port=3
  Out4 : Outport  Port=4
  Out5 : Outport  Port=5
  Out6 : Outport  Port=6
  Out7 : Outport  Port=7
  Out8 : Outport  Port=8
  wires:
  Relational Operator/1 -> Mux/1, Logical Operator/1
  [ref] -> Relational Operator3/1
  Sum2/1 -> Relational Operator2/2
  Repeating Sequence/1 -> Relational Operator/2, [Car], Sum/1
  Relational Operator1/1 -> Mux/3, Logical Operator1/1
  Relational Operator2/1 -> Mux1/1, Logical Operator2/1
  Constant/1 -> Sum/2
  Constant1/1 -> Sum2/2
  In1/1 -> [ref]
  Sum/1 -> Relational Operator1/2
  [ref] -> Relational Operator/1
  [Car] -> Sum3/1
  [ref] -> Relational Operator1/1
  [Car] -> Sum2/1
  Logical Operator/1 -> Mux/2
  Sum3/1 -> Relational Operator3/2
  Relational Operator3/1 -> Mux1/3, Logical Operator3/1
  [ref] -> Relational Operator2/1
  Constant2/1 -> Sum3/2
  Logical Operator1/1 -> Mux/4
  Logical Operator2/1 -> Mux1/2
  Logical Operator3/1 -> Mux1/4
  Mux/1 -> Multiport Switch1/3, Multiport Switch/2
  Mux1/1 -> Multiport Switch1/2, Multiport Switch/3
  [Cell_Sort_Freq] -> Sum1/1
  Constant3/1 -> Sum1/2
  Sum1/1 -> [Selector]
  Multiport Switch/1 -> Demux/1
  Multiport Switch1/1 -> Demux1/1
  Demux/1 -> Out1/1
  Demux/2 -> Out2/1
  Demux/3 -> Out3/1
  Demux/4 -> Out4/1
  Demux1/1 -> Out5/1
  Demux1/2 -> Out6/1
  Demux1/3 -> Out7/1
  Demux1/4 -> Out8/1
  [Selector] -> Multiport Switch/1
  [Selector] -> Multiport Switch1/1
  In2/1 -> [Cell_Sort_Freq]

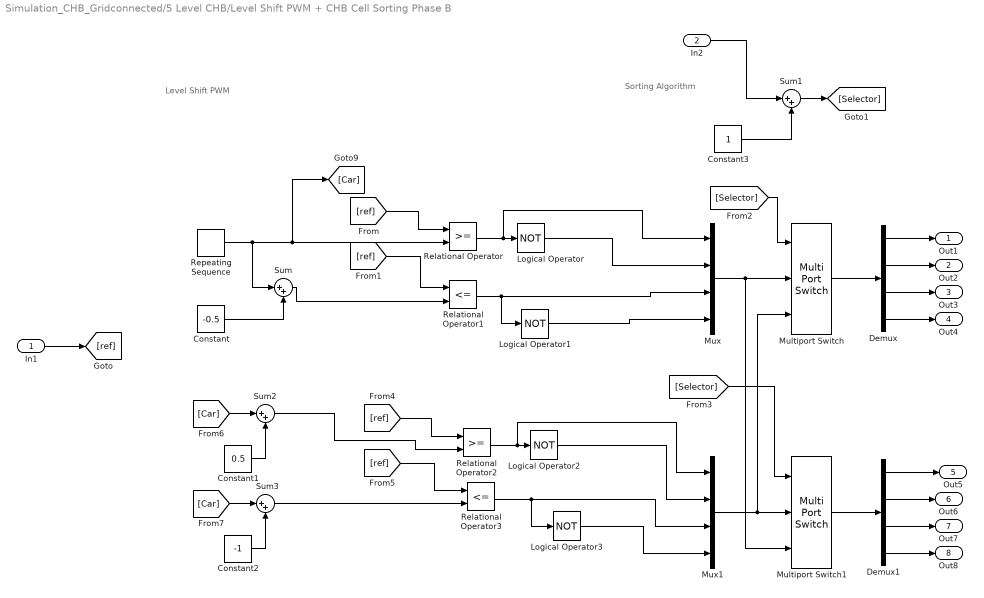
== system Simulation_CHB_Gridconnected/5 Level CHB/Level Shift PWM + CHB Cell Sorting Phase B ==
  note: Sorting Algorithm
  note: Level Shift PWM
  In1 : Inport
  In2 : Inport  Port=2
  Constant : Constant  Value=-0.5
  Constant1 : Constant  Value=0.5
  Constant2 : Constant  Value=-1
  Constant3 : Constant
  Demux : Demux
  Demux1 : Demux
  Logical Operator{,1..3} (4 alike) : Logic  Operator=NOT  AllPortsSameDT=off  OutDataTypeStr=boolean
  Multiport Switch : MultiPortSwitch  Inputs=2  SaturateOnIntegerOverflow=off  InputSameDT=off
  Multiport Switch1 : MultiPortSwitch  Inputs=2  SaturateOnIntegerOverflow=off  InputSameDT=off
  Mux : Mux
  Mux1 : Mux
  Relational Operator : RelationalOperator  OutDataTypeStr=boolean  RndMeth=Simplest  InputSameDT=off
  Relational Operator1 : RelationalOperator  Operator=<=  OutDataTypeStr=boolean  RndMeth=Simplest  InputSameDT=off
  Relational Operator2 : RelationalOperator  OutDataTypeStr=boolean  RndMeth=Simplest  InputSameDT=off
  Relational Operator3 : RelationalOperator  Operator=<=  OutDataTypeStr=boolean  RndMeth=Simplest  InputSameDT=off
  Repeating Sequence : simulink/Sources/Repeating Sequence  rep_seq_t=[0 0.5 1]/10000  rep_seq_y=[0 0.5 0]
  Sum{,1..3} (4 alike) : Sum  Inputs=|++
  Out1 : Outport
  Out2 : Outport  Port=2
  Out3 : Outport  Port=3
  Out4 : Outport  Port=4
  Out5 : Outport  Port=5
  Out6 : Outport  Port=6
  Out7 : Outport  Port=7
  Out8 : Outport  Port=8
  wires:
  [Selector] -> Multiport Switch1/1
  [Selector] -> Multiport Switch/1
  Demux1/4 -> Out8/1
  Demux1/3 -> Out7/1
  Demux1/2 -> Out6/1
  Demux1/1 -> Out5/1
  Demux/4 -> Out4/1
  Demux/3 -> Out3/1
  Demux/2 -> Out2/1
  Demux/1 -> Out1/1
  Multiport Switch1/1 -> Demux1/1
  Multiport Switch/1 -> Demux/1
  Sum1/1 -> [Selector]
  Constant3/1 -> Sum1/2
  In2/1 -> Sum1/1
  Mux1/1 -> Multiport Switch/3, Multiport Switch1/2
  Mux/1 -> Multiport Switch/2, Multiport Switch1/3
  Logical Operator3/1 -> Mux1/4
  Logical Operator2/1 -> Mux1/2
  Logical Operator1/1 -> Mux/4
  Constant2/1 -> Sum3/2
  [ref] -> Relational Operator2/1
  Relational Operator3/1 -> Logical Operator3/1, Mux1/3
  Sum3/1 -> Relational Operator3/2
  Logical Operator/1 -> Mux/2
  [Car] -> Sum2/1
  [ref] -> Relational Operator1/1
  [Car] -> Sum3/1
  [ref] -> Relational Operator/1
  Sum/1 -> Relational Operator1/2
  In1/1 -> [ref]
  Constant1/1 -> Sum2/2
  Constant/1 -> Sum/2
  Relational Operator2/1 -> Logical Operator2/1, Mux1/1
  Relational Operator1/1 -> Logical Operator1/1, Mux/3
  Repeating Sequence/1 -> Sum/1, [Car], Relational Operator/2
  Sum2/1 -> Relational Operator2/2
  [ref] -> Relational Operator3/1
  Relational Operator/1 -> Logical Operator/1, Mux/1

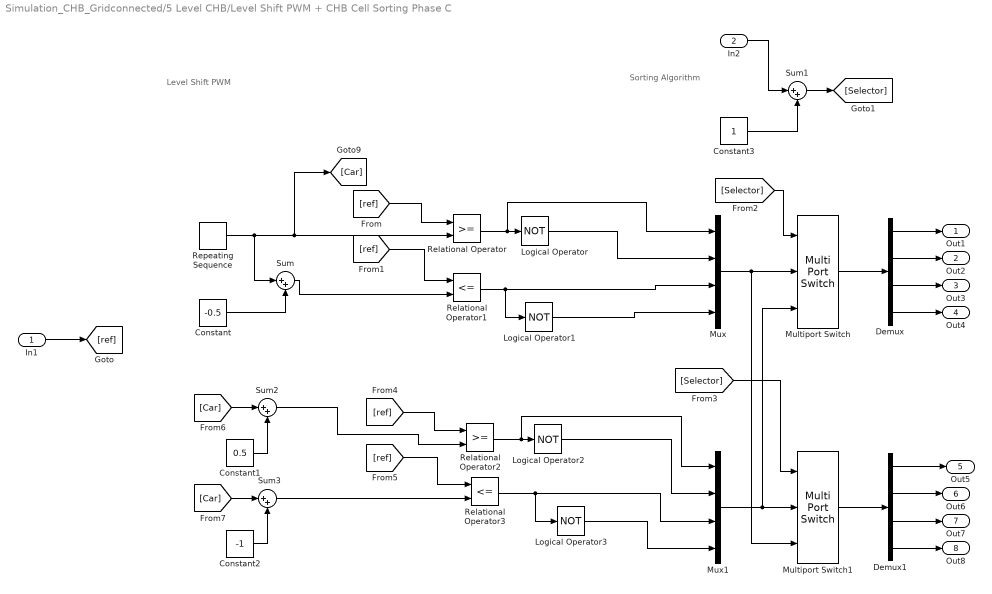
== system Simulation_CHB_Gridconnected/5 Level CHB/Level Shift PWM + CHB Cell Sorting Phase C ==
  note: Level Shift PWM
  note: Sorting Algorithm
  In1 : Inport
  In2 : Inport  Port=2
  Constant : Constant  Value=-0.5
  Constant1 : Constant  Value=0.5
  Constant2 : Constant  Value=-1
  Constant3 : Constant
  Demux : Demux
  Demux1 : Demux
  Logical Operator{,1..3} (4 alike) : Logic  Operator=NOT  AllPortsSameDT=off  OutDataTypeStr=boolean
  Multiport Switch : MultiPortSwitch  Inputs=2  SaturateOnIntegerOverflow=off  InputSameDT=off
  Multiport Switch1 : MultiPortSwitch  Inputs=2  SaturateOnIntegerOverflow=off  InputSameDT=off
  Mux : Mux
  Mux1 : Mux
  Relational Operator : RelationalOperator  OutDataTypeStr=boolean  RndMeth=Simplest  InputSameDT=off
  Relational Operator1 : RelationalOperator  Operator=<=  OutDataTypeStr=boolean  RndMeth=Simplest  InputSameDT=off
  Relational Operator2 : RelationalOperator  OutDataTypeStr=boolean  RndMeth=Simplest  InputSameDT=off
  Relational Operator3 : RelationalOperator  Operator=<=  OutDataTypeStr=boolean  RndMeth=Simplest  InputSameDT=off
  Repeating Sequence : simulink/Sources/Repeating Sequence  rep_seq_t=[0 0.5 1]/10000  rep_seq_y=[0 0.5 0]
  Sum{,1..3} (4 alike) : Sum  Inputs=|++
  Out1 : Outport
  Out2 : Outport  Port=2
  Out3 : Outport  Port=3
  Out4 : Outport  Port=4
  Out5 : Outport  Port=5
  Out6 : Outport  Port=6
  Out7 : Outport  Port=7
  Out8 : Outport  Port=8
  wires:
  Relational Operator/1 -> Mux/1, Logical Operator/1
  [ref] -> Relational Operator3/1
  Sum2/1 -> Relational Operator2/2
  Repeating Sequence/1 -> Relational Operator/2, [Car], Sum/1
  Relational Operator1/1 -> Mux/3, Logical Operator1/1
  Relational Operator2/1 -> Mux1/1, Logical Operator2/1
  Constant/1 -> Sum/2
  Constant1/1 -> Sum2/2
  In1/1 -> [ref]
  Sum/1 -> Relational Operator1/2
  [ref] -> Relational Operator/1
  [Car] -> Sum3/1
  [ref] -> Relational Operator1/1
  [Car] -> Sum2/1
  Logical Operator/1 -> Mux/2
  Sum3/1 -> Relational Operator3/2
  Relational Operator3/1 -> Mux1/3, Logical Operator3/1
  [ref] -> Relational Operator2/1
  Constant2/1 -> Sum3/2
  Logical Operator1/1 -> Mux/4
  Logical Operator2/1 -> Mux1/2
  Logical Operator3/1 -> Mux1/4
  Mux/1 -> Multiport Switch1/3, Multiport Switch/2
  Mux1/1 -> Multiport Switch1/2, Multiport Switch/3
  In2/1 -> Sum1/1
  Constant3/1 -> Sum1/2
  Sum1/1 -> [Selector]
  Multiport Switch/1 -> Demux/1
  Multiport Switch1/1 -> Demux1/1
  Demux/1 -> Out1/1
  Demux/2 -> Out2/1
  Demux/3 -> Out3/1
  Demux/4 -> Out4/1
  Demux1/1 -> Out5/1
  Demux1/2 -> Out6/1
  Demux1/3 -> Out7/1
  Demux1/4 -> Out8/1
  [Selector] -> Multiport Switch/1
  [Selector] -> Multiport Switch1/1

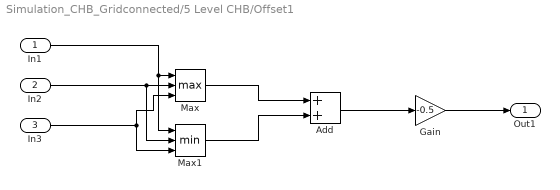
== system Simulation_CHB_Gridconnected/5 Level CHB/Offset1 ==
  In1 : Inport
  In2 : Inport  Port=2
  In3 : Inport  Port=3
  Add : Sum
  Gain : Gain  Gain=-0.5
  Max : MinMax  Function=max  Inputs=3
  Max1 : MinMax  Inputs=3
  Out1 : Outport
  wires:
  In2/1 -> Max1/2, Max/2
  In1/1 -> Max1/1, Max/1
  Max/1 -> Add/1
  In3/1 -> Max/3, Max1/3
  Gain/1 -> Out1/1
  Max1/1 -> Add/2
  Add/1 -> Gain/1
